simulink model "QBot2e_Path_Planning_Motion_Control"  (Simulink 10.1)
settings: Solver=ode1  StartTime=0.0  StopTime=inf  FixedStep=0.01  RelTol=1e-3  EnableMultiTasking=on
undefined symbols (not defined in the file or in its folder): HIL
libraries: quarc_library x8
settings Model: Creator=drmadill  LastModifiedBy=78253  SimulationMode=external  ExtModeTrigDuration=10000
settings SolverCC: PositivePriorityOrder=on
settings DataIOCC: LimitDataPoints=on  SignalLoggingSaveFormat=ModelDataLogs
settings OptimizationCC: ExpressionDepthLimit=2147483647  LifeSpan=auto
settings DebuggingCC: SolverPrmCheckMsg=warning  FcnCallInpInsideContextMsg=warning  StateNameClashWarn=warning
settings RTWCC: Description=QUARC Linux Raspberry Pi 3 Target  SystemTargetFile=quarc_linux_pi_3.tlc  TemplateMakefile=quarc_default_tmf
settings STFCustomTargetCC: TargetLibSuffix=.a  TargetPreCompLibLocation=C:\PROGRA~3\QUARC\lib\2018a\LINUX_~1\release  ConcurrentExecutionCompliant=on  SystemTargetFile=quarc_linux_pi_3.tlc
settings GRTTargetCC: TargetLibSuffix=.a  TargetPreCompLibLocation=C:\PROGRA~3\QUARC\lib\2018a\LINUX_~1\release  ParMdlRefBuildCompliant=off  CompOptLevelCompliant=off  MatFileLogging=off  CPPClassGenCompliant=off  UseToolchainInfoCompliant=off  ExtMode=on  ExtModeMexFile=quarc_comm  ExtModeMexArgs='-w -d /tmp -uri %u','tcpip://192.168.2.227:17001'
settings ConfigComp: CovSFcnEnable=off

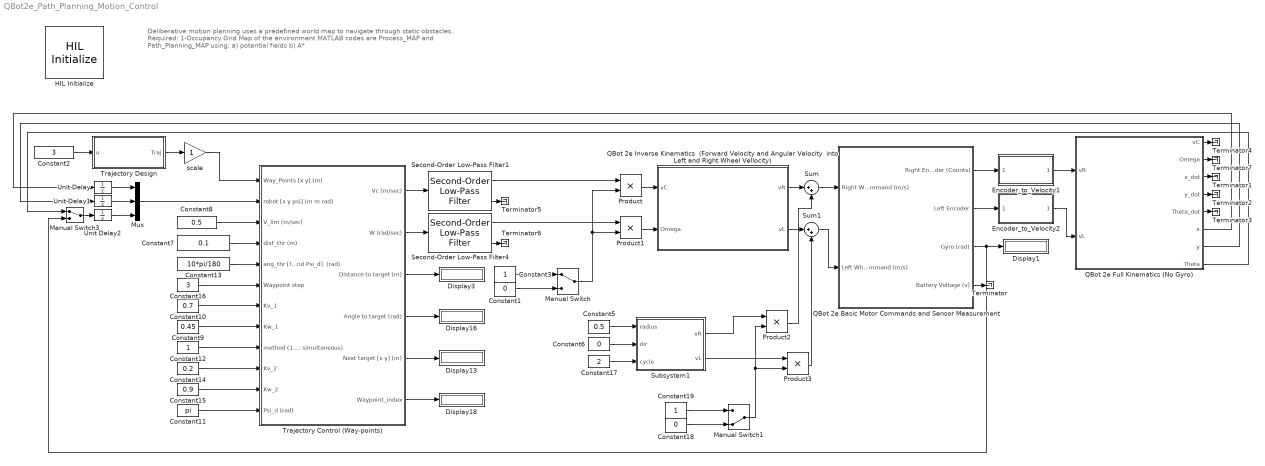
== system QBot2e_Path_Planning_Motion_Control ==
  note: Deliberative motion planning uses a predefined world map to navigate through static obstacles.
      |
      | Required:
      | 1-Occupancy Grid Map of the environment
      | MATLAB codes are Process_MAP and Path_Planning_MAP using:
      | a) potential fields
      | b) A*
  Constant1 : Constant  Value=0
  Constant10 : Constant  Value=0.7
  Constant11 : Constant  Value=pi
  Constant12 : Constant
  Constant13 : Constant  Value=10*pi/180
  Constant14 : Constant  Value=0.2
  Constant15 : Constant  Value=0.9
  Constant16 : Constant  Value=3
  Constant17 : Constant  Value=2
  Constant18 : Constant  Value=0
  Constant19 : Constant
  Constant2 : Constant  Value=3
  Constant3 : Constant
  Constant5 : Constant  Value=0.5
  Constant6 : Constant  Value=0
  Constant7 : Constant  Value=0.1
  Constant8 : Constant  Value=0.5
  Constant9 : Constant  Value=0.45
  Display{1,3,13,16,18} (5 alike) : Display
  Encoder_to_Velocity1 : Subsystem
  Encoder_to_Velocity2 : Subsystem
  HIL Initialize : quarc_library/Data Acquisition/Generic/Configuration/HIL Initialize  Priority=-99  object_name=HIL-1  board_type=qbot2e  board_number=0  board_options=pwm0_en=1;pwm0_pin=12;pwm1_en=1;pwm1_pin=13;  exclusive=off  active=off  hardware_clocks=[]  clock_modes=[]  initial_clock_frequencies=[]  set_clock_params_at_start=off  set_clock_params_at_switch_in=off  set_clock_frequencies_at_start=off  set_clock_frequencies_at_switch_in=off  analog_input_channels=[0:5]  analog_input_configurations=[]  analog_input_maximums=[16.5 3.3 3.3 3.3 3.3 3.3]  analog_input_minimums=[0 0 0 0 0 0]  set_analog_input_params_at_start=off  set_analog_input_params_at_switch_in=off  analog_output_channels=[]  analog_output_maximums=[]  analog_output_minimums=[]  initial_analog_outputs=[]  final_analog_outputs=[]  watchdog_analog_outputs=[]  set_analog_output_params_at_start=off  set_analog_output_params_at_switch_in=off  set_analog_outputs_at_start=off  set_analog_outputs_at_switch_in=off  set_analog_outputs_at_terminate=off  set_analog_outputs_at_switch_out=off  set_analog_outputs_on_watchdog=off  digital_input_channels=[28:58]  digital_output_channels=[28:31]  digital_output_configuration=[]  initial_digital_outputs=[0]  final_digital_outputs=[0]  watchdog_digital_outputs=[]  set_digital_output_params_at_start=off  set_digital_output_params_at_switch_in=off  set_digital_outputs_at_start=on  set_digital_outputs_at_switch_in=off  set_digital_outputs_at_terminate=on  set_digital_outputs_at_switch_out=off  set_digital_outputs_on_watchdog=off  encoder_channels=[0:1]  quadrature=[4]  encoder_filter_frequency=[]  initial_encoder_counts=[0]  set_encoder_params_at_start=on  set_encoder_params_at_switch_in=off  set_encoder_counts_at_start=on  set_encoder_counts_at_switch_in=off  pwm_channels=[0:1]  pwm_modes=0  pwm_frequency=100e6 / 4095  pwm_configuration=[0]  pwm_alignment=[0]  pwm_polarity=[1]  pwm_leading_deadband=[]  pwm_trailing_deadband=[]  initial_pwm_outputs=[0]  final_pwm_outputs=[0]  watchdog_pwm_outputs=[]  set_pwm_params_at_start=on  set_pwm_params_at_switch_in=off  set_pwm_outputs_at_start=on  set_pwm_outputs_at_switch_in=off  set_pwm_outputs_at_terminate=on  set_pwm_outputs_at_switch_out=off  set_pwm_outputs_on_watchdog=off  other_output_channels=[2000:2001 14000 16000]  initial_other_outputs=[0 0 0 7]  final_other_outputs=[0 0 0 7]  watchdog_other_outputs=[]  set_other_outputs_at_start=on  set_other_outputs_at_switch_in=off  set_other_outputs_at_terminate=on  set_other_outputs_at_switch_out=off  set_other_outputs_on_watchdog=off
  Manual Switch : ManualSwitch
  Manual Switch1 : ManualSwitch  CurrentSetting=0
  Manual Switch3 : ManualSwitch
  Mux : Mux  Inputs=[1 1 1]
  Product{,1..3} (4 alike) : Product  RndMeth=Zero
  QBot 2e Basic Motor Commands and Sensor Measurement : Subsystem
  QBot 2e Full Kinematics (No Gyro) : Subsystem
  QBot 2e Inverse Kinematics  (Forward Velocity and Angular Velocity  into Left and Right Wheel Vellocity) : Subsystem
  Second-Order Low-Pass Filter1 : quarc_library/Continuous/Second-Order Low-Pass Filter  params_source=Internal (dialog parameters)  input_width=30  input_zeta=1  input_init=0
  Second-Order Low-Pass Filter4 : quarc_library/Continuous/Second-Order Low-Pass Filter  params_source=Internal (dialog parameters)  input_width=60  input_zeta=1  input_init=0
  Subsystem1 : Subsystem
  Sum : Sum  Inputs=|++
  Sum1 : Sum  Inputs=|++
  Terminator{,1..7} (8 alike) : Terminator
  Trajectory Control (Way-points) : Subsystem
  Trajectory Design : Subsystem
  Unit Delay : UnitDelay  SampleTime=-1  HasFrameUpgradeWarning=on
  Unit Delay1 : UnitDelay  SampleTime=-1  HasFrameUpgradeWarning=on
  Unit Delay2 : UnitDelay  SampleTime=-1  HasFrameUpgradeWarning=on
  scale : Gain
  wires:
  Constant3/1 -> Manual Switch/1
  Constant1/1 -> Manual Switch/2
  QBot 2e Basic Motor Commands and Sensor Measurement/1(Right Encoder (Counts)) -> Encoder_to_Velocity1/1(Encoder)
  QBot 2e Basic Motor Commands and Sensor Measurement/2(Left Encoder) -> Encoder_to_Velocity2/1(Encoder)
  QBot 2e Basic Motor Commands and Sensor Measurement/3(Gyro (rad)) -> Display1/1, Manual Switch3/2
  QBot 2e Full Kinematics (No Gyro)/8(Theta) -> Manual Switch3/1
  Encoder_to_Velocity1/1(Velocity) -> QBot 2e Full Kinematics (No Gyro)/1(vR)
  Encoder_to_Velocity2/1(Velocity) -> QBot 2e Full Kinematics (No Gyro)/2(vL)
  Second-Order Low-Pass Filter1/1 -> Product/1
  Second-Order Low-Pass Filter4/1 -> Product1/1
  Product/1 -> QBot 2e Inverse Kinematics  (Forward Velocity and Angular Velocity  into Left and Right Wheel Vellocity)/1(vC)
  Product1/1 -> QBot 2e Inverse Kinematics  (Forward Velocity and Angular Velocity  into Left and Right Wheel Vellocity)/2(Omega)
  Manual Switch/1 -> Product/2, Product1/2
  QBot 2e Full Kinematics (No Gyro)/3(x_dot) -> Terminator1/1
  QBot 2e Full Kinematics (No Gyro)/4(y_dot) -> Terminator2/1
  QBot 2e Full Kinematics (No Gyro)/5(Theta_dot) -> Terminator3/1
  Constant8/1 -> Trajectory Control (Way-points)/3(V_lim (m/sec))
  Constant7/1 -> Trajectory Control (Way-points)/4(dist_thr (m))
  Constant13/1 -> Trajectory Control (Way-points)/5(ang_thr [for method 1 and Psi_d]  (rad))
  Constant16/1 -> Trajectory Control (Way-points)/6(Waypoint step)
  Trajectory Control (Way-points)/3(Distance to target (m)) -> Display3/1
  Mux/1 -> Trajectory Control (Way-points)/2(robot [x y psi] (m m rad))
  Unit Delay/1 -> Mux/1
  Unit Delay1/1 -> Mux/2
  Unit Delay2/1 -> Mux/3
  Constant10/1 -> Trajectory Control (Way-points)/7(Kv_1)
  Constant9/1 -> Trajectory Control (Way-points)/8(Kw_1)
  Trajectory Control (Way-points)/4(Angle to target (rad)) -> Display16/1
  scale/1 -> Trajectory Control (Way-points)/1(Way_Points [x y] (m))
  Trajectory Control (Way-points)/1(Vc (m/sec)) -> Second-Order Low-Pass Filter1/1
  Trajectory Control (Way-points)/2(W (rad/sec)) -> Second-Order Low-Pass Filter4/1
  Manual Switch3/1 -> Unit Delay2/1
  Trajectory Control (Way-points)/5(Next target [x y] (m)) -> Display13/1
  Constant14/1 -> Trajectory Control (Way-points)/10(Kv_2)
  Constant15/1 -> Trajectory Control (Way-points)/11(Kw_2)
  Constant12/1 -> Trajectory Control (Way-points)/9("method (1: sequential, 2: simultaneous)")
  Constant11/1 -> Trajectory Control (Way-points)/12(Psi_d (rad))
  Trajectory Control (Way-points)/6(Waypoint_index) -> Display18/1
  QBot 2e Full Kinematics (No Gyro)/6(x) -> Unit Delay/1
  QBot 2e Full Kinematics (No Gyro)/7(y) -> Unit Delay1/1
  Second-Order Low-Pass Filter1/2 -> Terminator5/1
  Second-Order Low-Pass Filter4/2 -> Terminator6/1
  QBot 2e Full Kinematics (No Gyro)/1(vC) -> Terminator4/1
  QBot 2e Full Kinematics (No Gyro)/2(Omega) -> Terminator7/1
  QBot 2e Basic Motor Commands and Sensor Measurement/4(Battery Voltage (v)) -> Terminator/1
  QBot 2e Inverse Kinematics  (Forward Velocity and Angular Velocity  into Left and Right Wheel Vellocity)/2(vL) -> Sum1/1
  QBot 2e Inverse Kinematics  (Forward Velocity and Angular Velocity  into Left and Right Wheel Vellocity)/1(vR) -> Sum/1
  Sum/1 -> QBot 2e Basic Motor Commands and Sensor Measurement/1(Right Wheel Command (m/s))
  Sum1/1 -> QBot 2e Basic Motor Commands and Sensor Measurement/2(Left Wheel Command (m/s))
  Constant5/1 -> Subsystem1/1(radius)
  Constant6/1 -> Subsystem1/2(dir)
  Constant17/1 -> Subsystem1/3(cycle)
  Constant18/1 -> Manual Switch1/2
  Constant19/1 -> Manual Switch1/1
  Manual Switch1/1 -> Product3/2, Product2/2
  Subsystem1/1(vR) -> Product2/1
  Subsystem1/2(vL) -> Product3/1
  Product2/1 -> Sum/2
  Product3/1 -> Sum1/2
  Constant2/1 -> Trajectory Design/1(u)
  Trajectory Design/1(Traj) -> scale/1

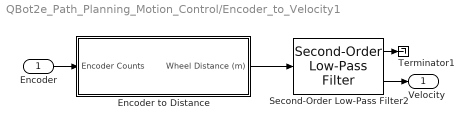
== system QBot2e_Path_Planning_Motion_Control/Encoder_to_Velocity1 ==
  Encoder : Inport
  Encoder to Distance : Subsystem
  Second-Order Low-Pass Filter2 : quarc_library/Continuous/Second-Order Low-Pass Filter  params_source=Internal (dialog parameters)  input_width=10  input_zeta=1  input_init=0
  Terminator1 : Terminator
  Velocity : Outport  VectorParamsAs1DForOutWhenUnconnected=off
  wires:
  Second-Order Low-Pass Filter2/1 -> Terminator1/1
  Encoder to Distance/1(Wheel Distance (m)) -> Second-Order Low-Pass Filter2/1
  Encoder/1 -> Encoder to Distance/1(Encoder Counts)
  Second-Order Low-Pass Filter2/2 -> Velocity/1

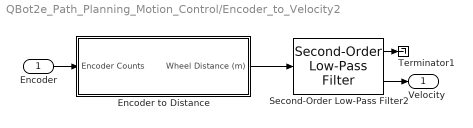
== system QBot2e_Path_Planning_Motion_Control/Encoder_to_Velocity2 ==
  Encoder : Inport
  Encoder to Distance : Subsystem
  Second-Order Low-Pass Filter2 : quarc_library/Continuous/Second-Order Low-Pass Filter  params_source=Internal (dialog parameters)  input_width=10  input_zeta=1  input_init=0
  Terminator1 : Terminator
  Velocity : Outport  VectorParamsAs1DForOutWhenUnconnected=off
  wires:
  Second-Order Low-Pass Filter2/2 -> Velocity/1
  Encoder/1 -> Encoder to Distance/1(Encoder Counts)
  Encoder to Distance/1(Wheel Distance (m)) -> Second-Order Low-Pass Filter2/1
  Second-Order Low-Pass Filter2/1 -> Terminator1/1

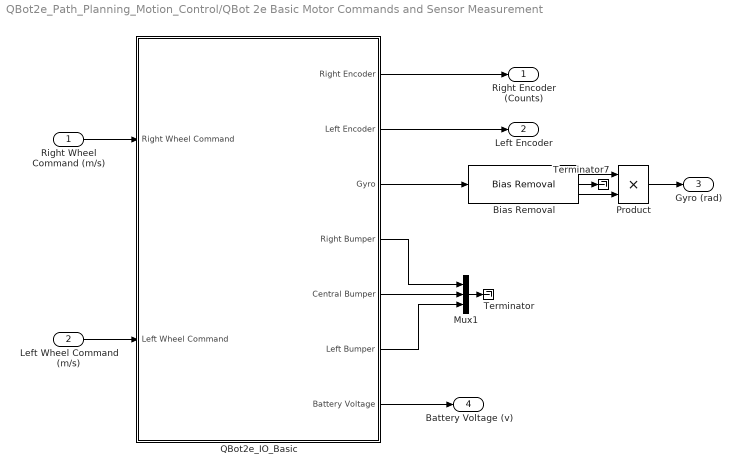
== system QBot2e_Path_Planning_Motion_Control/QBot 2e Basic Motor Commands and Sensor Measurement ==
  Right Wheel Command (m/s) : Inport
  Left Wheel Command (m/s) : Inport  Port=2
  Bias Removal : quarc_library/Discrete/Bias Removal  start_time=3  end_time=4  switch_id=0  sample_time=qc_get_step_size
      settings: SourceProductName=QUARC Targets
  Mux1 : Mux  Inputs=3
  Product : Product  RndMeth=Zero
  QBot2e_IO_Basic : Subsystem
  Terminator : Terminator
  Terminator7 : Terminator
  Right Encoder (Counts) : Outport  VectorParamsAs1DForOutWhenUnconnected=off
  Left Encoder : Outport  Port=2  VectorParamsAs1DForOutWhenUnconnected=off
  Gyro (rad) : Outport  Port=3  VectorParamsAs1DForOutWhenUnconnected=off
  Battery Voltage (v) : Outport  Port=4  VectorParamsAs1DForOutWhenUnconnected=off
  wires:
  QBot2e_IO_Basic/4(Right Bumper) -> Mux1/1
  QBot2e_IO_Basic/5(Central Bumper) -> Mux1/2
  QBot2e_IO_Basic/6(Left Bumper) -> Mux1/3
  Right Wheel Command (m/s)/1 -> QBot2e_IO_Basic/1(Right Wheel Command)
  Left Wheel Command (m/s)/1 -> QBot2e_IO_Basic/2(Left Wheel Command)
  QBot2e_IO_Basic/1(Right Encoder) -> Right Encoder (Counts)/1
  QBot2e_IO_Basic/2(Left Encoder) -> Left Encoder/1
  QBot2e_IO_Basic/7(Battery Voltage) -> Battery Voltage (v)/1
  Bias Removal/2 -> Terminator7/1
  Bias Removal/1 -> Product/1
  Bias Removal/3 -> Product/2
  Product/1 -> Gyro (rad)/1
  QBot2e_IO_Basic/3(Gyro) -> Bias Removal/1
  Mux1/1 -> Terminator/1

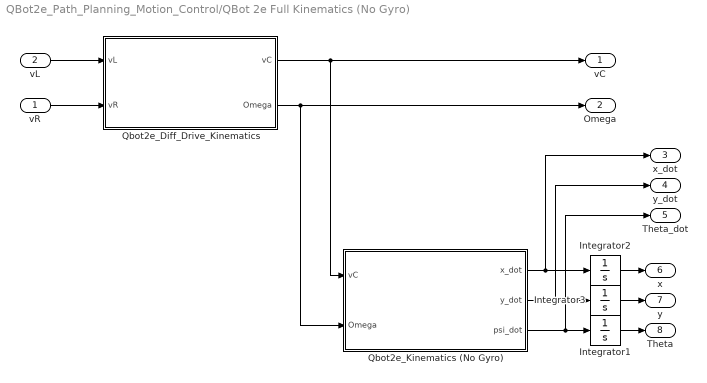
== system QBot2e_Path_Planning_Motion_Control/QBot 2e Full Kinematics (No Gyro) ==
  vR : Inport
  vL : Inport  Port=2
  Integrator1 : Integrator
  Integrator2 : Integrator
  Integrator3 : Integrator
  Qbot2e_Diff_Drive_Kinematics : Subsystem
  Qbot2e_Kinematics (No Gyro) : Subsystem
  vC : Outport  VectorParamsAs1DForOutWhenUnconnected=off
  Omega : Outport  Port=2  VectorParamsAs1DForOutWhenUnconnected=off
  x_dot : Outport  Port=3  VectorParamsAs1DForOutWhenUnconnected=off
  y_dot : Outport  Port=4  VectorParamsAs1DForOutWhenUnconnected=off
  Theta_dot : Outport  Port=5  VectorParamsAs1DForOutWhenUnconnected=off
  x : Outport  Port=6  VectorParamsAs1DForOutWhenUnconnected=off
  y : Outport  Port=7  VectorParamsAs1DForOutWhenUnconnected=off
  Theta : Outport  Port=8  VectorParamsAs1DForOutWhenUnconnected=off
  wires:
  Integrator1/1 -> Theta/1
  Qbot2e_Kinematics (No Gyro)/3(psi_dot) -> Theta_dot/1, Integrator1/1
  Qbot2e_Kinematics (No Gyro)/1(x_dot) -> x_dot/1, Integrator2/1
  Qbot2e_Kinematics (No Gyro)/2(y_dot) -> y_dot/1, Integrator3/1
  Qbot2e_Diff_Drive_Kinematics/1(vC) -> Qbot2e_Kinematics (No Gyro)/1(vC), vC/1
  vL/1 -> Qbot2e_Diff_Drive_Kinematics/1(vL)
  vR/1 -> Qbot2e_Diff_Drive_Kinematics/2(vR)
  Integrator2/1 -> x/1
  Integrator3/1 -> y/1
  Qbot2e_Diff_Drive_Kinematics/2(Omega) -> Qbot2e_Kinematics (No Gyro)/2(Omega), Omega/1

== system QBot2e_Path_Planning_Motion_Control/QBot 2e Inverse Kinematics  (Forward Velocity and Angular Velocity  into Left and Right Wheel Vellocity) ==
  vC : Inport
  Omega : Inport  Port=2
  Qbot2e_Inverse_Kinematics  (Forward Velocity and Angular Velocity into Left and Right Wheel Vellocity) : MATLAB Function  TreatAsAtomicUnit=on
  vR : Outport  VectorParamsAs1DForOutWhenUnconnected=off
  vL : Outport  Port=2  VectorParamsAs1DForOutWhenUnconnected=off
  wires:
  Qbot2e_Inverse_Kinematics  (Forward Velocity and Angular Velocity into Left and Right Wheel Vellocity)/2(vL) -> vL/1
  Omega/1 -> Qbot2e_Inverse_Kinematics  (Forward Velocity and Angular Velocity into Left and Right Wheel Vellocity)/2(Omega)
  Qbot2e_Inverse_Kinematics  (Forward Velocity and Angular Velocity into Left and Right Wheel Vellocity)/1(vR) -> vR/1
  vC/1 -> Qbot2e_Inverse_Kinematics  (Forward Velocity and Angular Velocity into Left and Right Wheel Vellocity)/1(vC)

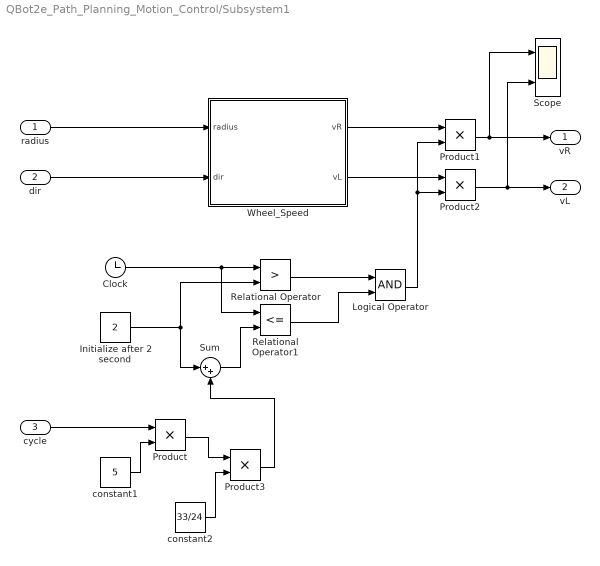
== system QBot2e_Path_Planning_Motion_Control/Subsystem1 ==
  radius : Inport
  dir : Inport  Port=2
  cycle : Inport  Port=3
  Clock : Clock
  Initialize after 2 second : Constant  Value=2
  Logical Operator : Logic  AllPortsSameDT=off  OutDataTypeStr=boolean
  Product{,1..3} (4 alike) : Product
  Relational Operator : RelationalOperator  Operator=>  OutDataTypeStr=boolean  RndMeth=Simplest
  Relational Operator1 : RelationalOperator  Operator=<=  OutDataTypeStr=boolean  RndMeth=Simplest
  Scope : Scope  NumInputPorts=2
  Sum : Sum  Inputs=|++
  Wheel_Speed : MATLAB Function  TreatAsAtomicUnit=on
  constant1 : Constant  Value=5
  constant2 : Constant  Value=33/24
  vR : Outport
  vL : Outport  Port=2
  wires:
  Sum/1 -> Relational Operator1/2
  Clock/1 -> Relational Operator1/1, Relational Operator/1
  Product2/1 -> Scope/2, vL/1
  Product1/1 -> Scope/1, vR/1
  Wheel_Speed/2(vL) -> Product2/1
  Relational Operator1/1 -> Logical Operator/2
  dir/1 -> Wheel_Speed/2(dir)
  cycle/1 -> Product/1
  Relational Operator/1 -> Logical Operator/1
  constant1/1 -> Product/2
  radius/1 -> Wheel_Speed/1(radius)
  Logical Operator/1 -> Product2/2, Product1/2
  Initialize after 2 second/1 -> Sum/1, Relational Operator/2
  Wheel_Speed/1(vR) -> Product1/1
  Product/1 -> Product3/1
  constant2/1 -> Product3/2
  Product3/1 -> Sum/2

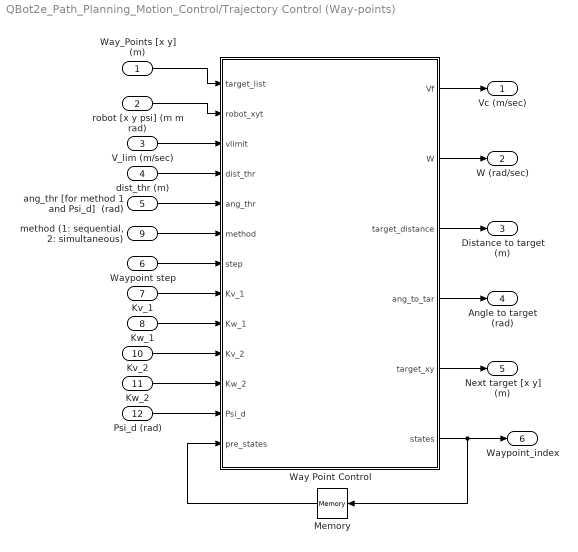
== system QBot2e_Path_Planning_Motion_Control/Trajectory Control (Way-points) ==
  Way_Points [x y] (m) : Inport
  robot [x y psi] (m m rad) : Inport  Port=2
  V_lim (m/sec) : Inport  Port=3
  dist_thr (m) : Inport  Port=4
  ang_thr [for method 1 and Psi_d]  (rad) : Inport  Port=5
  Waypoint step : Inport  Port=6
  Kv_1 : Inport  Port=7
  Kw_1 : Inport  Port=8
  "method (1: sequential, 2: simultaneous)" : Inport  Port=9
  Kv_2 : Inport  Port=10
  Kw_2 : Inport  Port=11
  Psi_d (rad) : Inport  Port=12
  Memory : Memory  InitialCondition=[0]
  Way Point Control : MATLAB Function  TreatAsAtomicUnit=on
  Vc (m/sec) : Outport  VectorParamsAs1DForOutWhenUnconnected=off
  W (rad/sec) : Outport  Port=2  VectorParamsAs1DForOutWhenUnconnected=off
  Distance to target (m) : Outport  Port=3  VectorParamsAs1DForOutWhenUnconnected=off
  Angle to target (rad) : Outport  Port=4  VectorParamsAs1DForOutWhenUnconnected=off
  Next target [x y] (m) : Outport  Port=5  VectorParamsAs1DForOutWhenUnconnected=off
  Waypoint_index : Outport  Port=6  VectorParamsAs1DForOutWhenUnconnected=off
  wires:
  Memory/1 -> Way Point Control/13(pre_states)
  Way Point Control/6(states) -> Memory/1, Waypoint_index/1
  Way_Points [x y] (m)/1 -> Way Point Control/1(target_list)
  Way Point Control/1(Vf) -> Vc (m/sec)/1
  robot [x y psi] (m m rad)/1 -> Way Point Control/2(robot_xyt)
  V_lim (m/sec)/1 -> Way Point Control/3(vlimit)
  Way Point Control/2(W) -> W (rad/sec)/1
  dist_thr (m)/1 -> Way Point Control/4(dist_thr)
  Way Point Control/3(target_distance) -> Distance to target (m)/1
  ang_thr [for method 1 and Psi_d]  (rad)/1 -> Way Point Control/5(ang_thr)
  Way Point Control/4(ang_to_tar) -> Angle to target (rad)/1
  Waypoint step/1 -> Way Point Control/7(step)
  Kv_1/1 -> Way Point Control/8(Kv_1)
  Way Point Control/5(target_xy) -> Next target [x y] (m)/1
  Kw_1/1 -> Way Point Control/9(Kw_1)
  "method (1: sequential, 2: simultaneous)"/1 -> Way Point Control/6(method)
  Kv_2/1 -> Way Point Control/10(Kv_2)
  Kw_2/1 -> Way Point Control/11(Kw_2)
  Psi_d (rad)/1 -> Way Point Control/12(Psi_d)

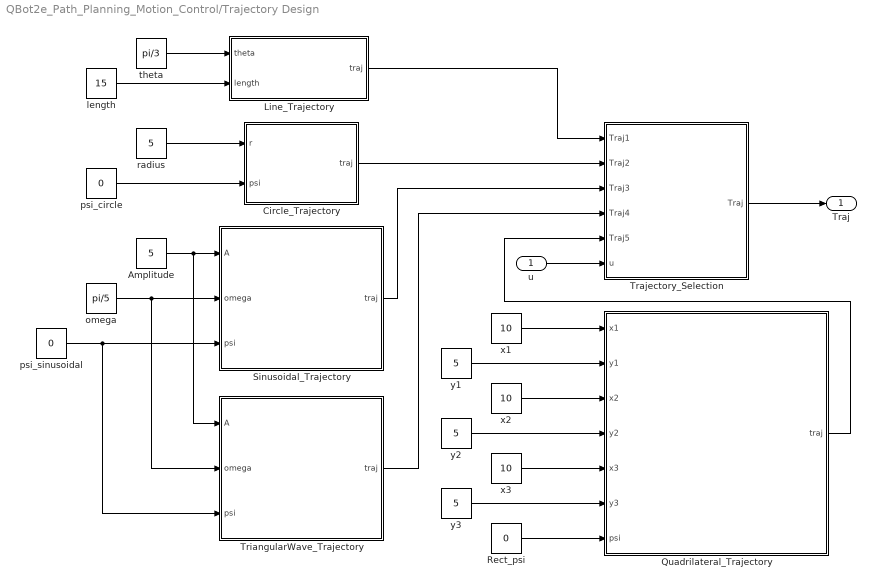
== system QBot2e_Path_Planning_Motion_Control/Trajectory Design ==
  u : Inport
  Amplitude : Constant  Value=5
  Circle_Trajectory : MATLAB Function  TreatAsAtomicUnit=on
  Line_Trajectory : MATLAB Function  TreatAsAtomicUnit=on
  "Quadrilateral_Trajectory " : MATLAB Function  TreatAsAtomicUnit=on
  Rect_psi : Constant  Value=0
  Sinusoidal_Trajectory : MATLAB Function  TreatAsAtomicUnit=on
  Trajectory_Selection : MATLAB Function  TreatAsAtomicUnit=on
  TriangularWave_Trajectory : MATLAB Function  TreatAsAtomicUnit=on
  length : Constant  Value=15
  omega : Constant  Value=pi/5
  psi_circle : Constant  Value=0
  psi_sinusoidal : Constant  Value=0
  radius : Constant  Value=5
  theta : Constant  Value=pi/3
  x1 : Constant  Value=10
  x2 : Constant  Value=10
  x3 : Constant  Value=10
  y1 : Constant  Value=5
  y2 : Constant  Value=5
  y3 : Constant  Value=5
  Traj : Outport
  wires:
  Trajectory_Selection/1(Traj) -> Traj/1
  Circle_Trajectory/1(traj) -> Trajectory_Selection/2(Traj2)
  psi_sinusoidal/1 -> TriangularWave_Trajectory/3(psi), Sinusoidal_Trajectory/3(psi)
  Amplitude/1 -> Sinusoidal_Trajectory/1(A), TriangularWave_Trajectory/1(A)
  omega/1 -> TriangularWave_Trajectory/2(omega), Sinusoidal_Trajectory/2(omega)
  Sinusoidal_Trajectory/1(traj) -> Trajectory_Selection/3(Traj3)
  theta/1 -> Line_Trajectory/1(theta)
  length/1 -> Line_Trajectory/2(length)
  psi_circle/1 -> Circle_Trajectory/2(psi)
  radius/1 -> Circle_Trajectory/1(r)
  Line_Trajectory/1(traj) -> Trajectory_Selection/1(Traj1)
  u/1 -> Trajectory_Selection/6(u)
  x1/1 -> "Quadrilateral_Trajectory "/1(x1)
  y1/1 -> "Quadrilateral_Trajectory "/2(y1)
  Rect_psi/1 -> "Quadrilateral_Trajectory "/7(psi)
  x2/1 -> "Quadrilateral_Trajectory "/3(x2)
  y2/1 -> "Quadrilateral_Trajectory "/4(y2)
  x3/1 -> "Quadrilateral_Trajectory "/5(x3)
  y3/1 -> "Quadrilateral_Trajectory "/6(y3)
  "Quadrilateral_Trajectory "/1(traj) -> Trajectory_Selection/5(Traj5)
  TriangularWave_Trajectory/1(traj) -> Trajectory_Selection/4(Traj4)

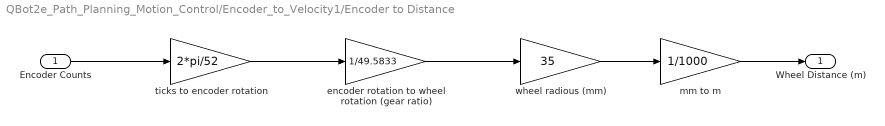
== system QBot2e_Path_Planning_Motion_Control/Encoder_to_Velocity1/Encoder to Distance ==
  Encoder Counts : Inport
  " encoder rotation to wheel rotation (gear ratio)" : Gain  Gain=1/49.5833
  mm to m : Gain  Gain=1/1000
  ticks to encoder rotation : Gain  Gain=2*pi/52
  wheel radious (mm) : Gain  Gain=35
  Wheel Distance (m) : Outport  VectorParamsAs1DForOutWhenUnconnected=off
  wires:
  Encoder Counts/1 -> ticks to encoder rotation/1
  ticks to encoder rotation/1 -> " encoder rotation to wheel rotation (gear ratio)"/1
  " encoder rotation to wheel rotation (gear ratio)"/1 -> wheel radious (mm)/1
  wheel radious (mm)/1 -> mm to m/1
  mm to m/1 -> Wheel Distance (m)/1

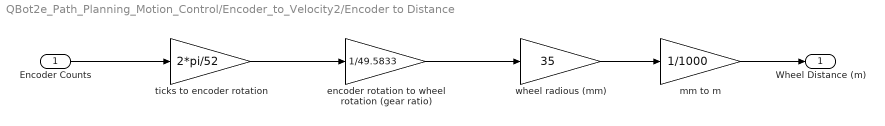
== system QBot2e_Path_Planning_Motion_Control/Encoder_to_Velocity2/Encoder to Distance ==
  Encoder Counts : Inport
  " encoder rotation to wheel rotation (gear ratio)" : Gain  Gain=1/49.5833
  mm to m : Gain  Gain=1/1000
  ticks to encoder rotation : Gain  Gain=2*pi/52
  wheel radious (mm) : Gain  Gain=35
  Wheel Distance (m) : Outport  VectorParamsAs1DForOutWhenUnconnected=off
  wires:
  mm to m/1 -> Wheel Distance (m)/1
  wheel radious (mm)/1 -> mm to m/1
  " encoder rotation to wheel rotation (gear ratio)"/1 -> wheel radious (mm)/1
  ticks to encoder rotation/1 -> " encoder rotation to wheel rotation (gear ratio)"/1
  Encoder Counts/1 -> ticks to encoder rotation/1

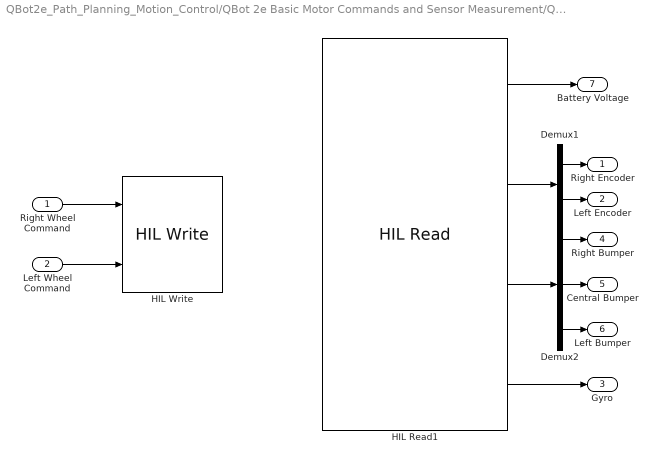
== system QBot2e_Path_Planning_Motion_Control/QBot 2e Basic Motor Commands and Sensor Measurement/QBot2e_IO_Basic ==
  Right Wheel Command : Inport
  Left Wheel Command : Inport  Port=2
  Demux1 : Demux  Outputs=2
  Demux2 : Demux  Outputs=3
  HIL Read1 : quarc_library/Data Acquisition/Generic/Immediate I//O/HIL Read  object_name=HIL-1  analog_channels=[0]  encoder_channels=[0:1]  digital_channels=[28:30]  other_channels=[1002]  sample_time=qc_get_step_size  active=on  vector_output=on  data_type_mode=Inherit via back propagation  encoder_data_type=double  digital_data_type=boolean
  HIL Write : quarc_library/Data Acquisition/Generic/Immediate I//O/HIL Write  object_name=HIL-1  analog_channels=[]  pwm_channels=[]  digital_channels=[]  other_channels=[2000:2001]  sample_time=-1  active=on  vector_input=off
  Right Encoder : Outport  VectorParamsAs1DForOutWhenUnconnected=off
  Left Encoder : Outport  Port=2  VectorParamsAs1DForOutWhenUnconnected=off
  Gyro : Outport  Port=3  VectorParamsAs1DForOutWhenUnconnected=off
  Right Bumper : Outport  Port=4  VectorParamsAs1DForOutWhenUnconnected=off
  Central Bumper : Outport  Port=5  VectorParamsAs1DForOutWhenUnconnected=off
  Left Bumper : Outport  Port=6  VectorParamsAs1DForOutWhenUnconnected=off
  Battery Voltage : Outport  Port=7  VectorParamsAs1DForOutWhenUnconnected=off
  wires:
  HIL Read1/1 -> Battery Voltage/1
  HIL Read1/3 -> Demux2/1
  HIL Read1/4 -> Gyro/1
  Demux1/1 -> Right Encoder/1
  Demux1/2 -> Left Encoder/1
  Right Wheel Command/1 -> HIL Write/1
  Left Wheel Command/1 -> HIL Write/2
  HIL Read1/2 -> Demux1/1
  Demux2/1 -> Right Bumper/1
  Demux2/2 -> Central Bumper/1
  Demux2/3 -> Left Bumper/1

== system QBot2e_Path_Planning_Motion_Control/QBot 2e Full Kinematics (No Gyro)/Qbot2e_Diff_Drive_Kinematics ==
  vL : Inport
  vR : Inport  Port=2
  Qbot2_Diff_Drive_Kinematics : MATLAB Function  TreatAsAtomicUnit=on
  vC : Outport  VectorParamsAs1DForOutWhenUnconnected=off
  Omega : Outport  Port=2  VectorParamsAs1DForOutWhenUnconnected=off
  wires:
  vL/1 -> Qbot2_Diff_Drive_Kinematics/1(vL)
  Qbot2_Diff_Drive_Kinematics/1(vC) -> vC/1
  vR/1 -> Qbot2_Diff_Drive_Kinematics/2(vR)
  Qbot2_Diff_Drive_Kinematics/2(Omega) -> Omega/1

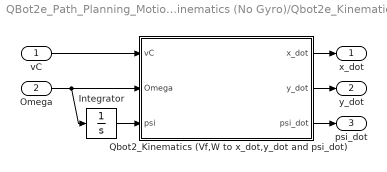
== system QBot2e_Path_Planning_Motion_Control/QBot 2e Full Kinematics (No Gyro)/Qbot2e_Kinematics (No Gyro) ==
  vC : Inport
  Omega : Inport  Port=2
  Integrator : Integrator
  Qbot2_Kinematics (Vf,W to x_dot,y_dot and psi_dot) : MATLAB Function  TreatAsAtomicUnit=on
  x_dot : Outport  VectorParamsAs1DForOutWhenUnconnected=off
  y_dot : Outport  Port=2  VectorParamsAs1DForOutWhenUnconnected=off
  psi_dot : Outport  Port=3  VectorParamsAs1DForOutWhenUnconnected=off
  wires:
  Qbot2_Kinematics (Vf,W to x_dot,y_dot and psi_dot)/3(psi_dot) -> psi_dot/1
  Integrator/1 -> Qbot2_Kinematics (Vf,W to x_dot,y_dot and psi_dot)/3(psi)
  vC/1 -> Qbot2_Kinematics (Vf,W to x_dot,y_dot and psi_dot)/1(vC)
  Qbot2_Kinematics (Vf,W to x_dot,y_dot and psi_dot)/1(x_dot) -> x_dot/1
  Omega/1 -> Integrator/1, Qbot2_Kinematics (Vf,W to x_dot,y_dot and psi_dot)/2(Omega)
  Qbot2_Kinematics (Vf,W to x_dot,y_dot and psi_dot)/2(y_dot) -> y_dot/1

== matlab function Trajectory Design/Circle_Trajectory ==
  data: traj output double; r input double; psi input double
function traj = Cir_Traj(r, psi)
% First we only care about the specific circle that satisfies
% x^2 + (y-r)^2 = r^2, where r is the radius of the circle.
% And in the polar coordinate system, it is:
% ρ = 2*r*sin(θ), where θ is between 0 and π.

% From the start point to the end point, there are N steps.
% Thus we divide π into N segments, that is, for the i th point sampled in
% the trajectory, its polar coordinate (ρi,θi) = (2*r*sin(θi), θi),
% where θi = (π/N)*(i-1).
% Finally, change the polar coordinate back to the Cartesian (xi, yi).

% Then, if the circle is rotated around the origin by ψ counterclockwise,
% we just do a coordinate transformation.

traj = zeros(20, 2);   % initialize

for i = 1 : 20
    theta_i = (pi/19) * (i-1);
    rou_i = 2 * r * sin(theta_i);
    px_t = rou_i * cos(theta_i);
    py_t = rou_i * sin(theta_i);
    % coordinate transformation when the circle is rotated by psi
    traj(i,1) = px_t * cos(psi) - py_t * sin(psi);
    traj(i,2) = px_t * sin(psi) + py_t * cos(psi);
end

== matlab function QBot 2e Full Kinematics (No Gyro)/Qbot2e_Diff_Drive_Kinematics/Qbot2_Diff_Drive_Kinematics ==
  data: vL input double; vC output double; vR input double; Omega output double
function [vC,Omega] = fcn(vL,vR)
%#codegen

d= 0.235;

vC=0.5*(vL+vR);
Omega=(1/d)*(vR-vL);

== matlab function QBot 2e Full Kinematics (No Gyro)/Qbot2e_Kinematics (No Gyro)/Qbot2_Kinematics (Vf,W to x_dot,y_dot and psi_dot) ==
  data: vC input double; x_dot output double; Omega input double; y_dot output double; psi input double; psi_dot output double
function [x_dot,y_dot,psi_dot] = fcn(vC,Omega,psi)
%#codegen


x_dot=cos(psi)*vC;
y_dot=sin(psi)*vC;
psi_dot= Omega;

== matlab function Trajectory Control (Way-points)/Way Point Control ==
  data: target_list input double; robot_xyt input double; vlimit input double; dist_thr input double; ang_thr input double; method input double; step input double; Kv_1 input double; Kw_1 input double; Kv_2 input double; Kw_2 input double; Psi_d input double; Vf output double; W output double; target_distance output double; ang_to_tar output double; target_xy output double; states output double; pre_states input double
function [Vf, W, target_distance, ang_to_tar, target_xy, states] = ...
    WaypointControl(target_list, robot_xyt, vlimit, ...
    dist_thr, ang_thr, method, step, Kv_1, Kw_1, Kv_2, Kw_2, Psi_d, pre_states)

% Initialize output variables

 Vf=0;
 W=0;
 finished_path_flag=0; 
 
 persistent Vf_1 end_flag;
 
 if isempty(Vf_1)
     Vf_1=0;
 end
 if isempty(end_flag)
    end_flag = 0;
 end
states = pre_states;



rx = robot_xyt(1);
ry = robot_xyt(2);
rtheta = check_angle(robot_xyt(3));
target_xy = [rx ry];
[n xy] = size(target_list);
if n==2 && xy==1
    target_xy = [target_list(1,1) target_list(2,1)];
    n = 1;
else
    for i=1:n
        if states(1) == i
            for j=1:xy
                target_xy(j) = target_list(i, j);
            end
        end
    end
end

tx = target_xy(1);
ty = target_xy(2);
target_distance = find_dist(rx, ry, tx, ty);
ang_to_tar= find_theta(rx, ry, rtheta, tx, ty);

if ((states(1) == n) && (target_distance <= dist_thr))  %|| states(1) == -1
% %        states(1) = -1;
       % right_vel = int16(0);
       % left_vel = int16(0);
%  %       target_distance = 0;
        Vf=0;
        W=0;
        
       if (end_flag == 1) && (target_distance <= dist_thr) % after all waypoints, psi will be adjusted to psi_d 
            [Vf, W] = ClosedLoop_Sequential(0, check_angle(check_angle(Psi_d)-check_angle(rtheta)), vlimit, ang_thr, dist_thr, Kv_1, Kw_1, Vf_1); 
             Vf_1=Vf;
       end
        
   
else
    
    if (target_distance <= dist_thr) && (end_flag==0)
            states(1) = pre_states(1) + step;%1;
      if( pre_states(1)>0 )      
         while (abs((target_list(states(1),1))-(target_list(pre_states(1),1)))<2*dist_thr) && (abs((target_list(states(1),2))-(target_list(pre_states(1),2)))<2*dist_thr)
             if (states(1)<=(n-step))
                 states(1) = states(1) + step;%1;
             else
                 states(1)=n;
             end
         end
      else
          states(1)=states(1)+step;
      end
         if states(1) >= n 
            states(1) = n;
            end_flag=1;
         end
        
               
  %  elseif (end_flag == 1) && (target_distance <= dist_thr) % after all waypoints, psi will be adjusted to psi_d 
  %          [Vf, W] = ClosedLoop_Sequential(0, check_angle(check_angle(Psi_d)-check_angle(rtheta)), vlimit, ang_thr, dist_thr, Kv_1, Kw_1, Vf_1); 
  %           Vf_1=Vf;
    else
        
        
            if method == 2
                [Vf, W] = ClosedLoop_Both(target_distance,  ang_to_tar, vlimit, Kv_2, Kw_2);    
            else
    %            [right_vel, left_vel] = rotate_and_go(ang_to_tar, vlimit, ang_thr);
                [Vf, W] = ClosedLoop_Sequential(target_distance,  ang_to_tar, vlimit, ang_thr, dist_thr, Kv_1, Kw_1, Vf_1); 
                Vf_1=Vf;
            end
                 
    end
end


return;

%--------------------------------------------------------------------------
function [y] = check_angle(x)
y = x;
if x > pi
    y = x - 2*pi;
elseif x < -pi
    y = x + 2*pi;
end
return;
% -------------------------------------------------------------------------
function dist = find_dist(rx, ry, tx, ty)
dist = sqrt((rx-tx)^2 + (ry-ty)^2);
return;
% -------------------------------------------------------------------------
function [theta]= find_theta(rx, ry, rtheta, tx, ty)

X = tx - rx;
Y = ty - ry;
theta = atan2(Y, X);
theta = check_angle(check_angle(theta)-check_angle(rtheta));

return;
% -------------------------------------------------------------------------

function [Vf, W] = ClosedLoop_Both(dist, theta, vlimit, Kv,Kw)

d = 0.23;
vmax = vlimit;
wmax = (2*vmax);
W = Kw*theta;

%if abs(theta)<pi
Vf = Kv*dist;
%else
%    Vf=0;
%end

w_sign = sign(W);
if abs(W) > wmax
    W = w_sign*wmax;
end
if abs(Vf)> vlimit
    Vf = abs(Vf)*vlimit;
end

return;

function [Vf, W] = ClosedLoop_Sequential(dist, theta, vlimit, ang_thr, dist_thr, Kv, Kw, Vf_1)

d = 0.23;
vmax = vlimit;
wmax = (2*vmax);

if (((abs(theta) > ang_thr))  && (Vf_1<0.01)) || (abs(theta) > 5*ang_thr) % once rotated, then moves. once started moving, it won't turn unless the heading is too off target or have reached the previous target.
        W=Kw*theta;
        Vf=0;
        if abs(W)> wmax
            W=sign(theta)*wmax;
        end
else
        Vf=Kv*dist;
       
        if abs(Vf)>vlimit
            Vf=sign(Vf)*vlimit;
        end
       % if (abs(theta) > 2*ang_thr)
       %   W=Kw*theta;
       %   Vf=0.4*Vf;
       % else
       W=0;
       % end
       % if abs(W)> wmax
       %     W=sign(theta)*wmax;
       % end
        
end

return;

%{
function [vr, vl] = solve_inv_kin(dist, theta, vlimit, delta_t)

d = 0.23;
vmax = vlimit(2);
wmax = (2*vmax)/d;
w = theta/delta_t;
w_sign = sign(w);
if abs(w) > wmax
    w = w_sign*wmax;
    vr = int16(round((d*w)/2));
    vl = int16(-vr);
else
    v = dist/delta_t;
    vr_tmp = (2*v + d*w)/2;
    vl_tmp = 2*v - vr_tmp;
    
    max_of_vrvl = abs(max(vr_tmp, vl_tmp));
    if max_of_vrvl > vmax
        vr_tmp = (vr_tmp/max_of_vrvl)*vmax;
        vl_tmp = (vl_tmp/max_of_vrvl)*vmax;
    end
    vr = int16(vr_tmp);
    vl = int16(vl_tmp);

end


return;
%}

%{
% -------------------------------------------------------------------------
function [vr, vl] = rotate_and_go(theta, vlimit, ang_thr)

if abs(theta) > ang_thr
    if theta >= 0
        vr = int16(vlimit(1));
        vl = int16(-vlimit(1));
    else
        vr = int16(-vlimit(1));
        vl = int16(vlimit(1));
    end
else
        vr = int16(vlimit(2));
        vl = int16(vlimit(2));
end

return;
% -------------------------------------------------------------------------
%}

== matlab function Trajectory Design/Line_Trajectory ==
  data: traj output double; theta input double; length input double
function traj = Line_Traj(theta, length)
% theta is the dip angle by the x-axis, thus the slope k = tan(theta).
% theta is radian instead of degree.

% length is the length of the line trajectory.

traj = zeros(20, 2);   % initialize

length_x = length * cos(theta);
length_y = length * sin(theta);

for i = 1 : 20
    traj(i,1) = length_x/20 * (i-1);
    traj(i,2) = length_y/20 * (i-1);
end

== matlab function Trajectory Design/Sinusoidal_Trajectory ==
  data: traj output double; A input double; omega input double; psi input double
function traj = Sin_Traj(A, omega, psi)
% We always and only focus on the sinusoidal curve whose phase is 0.

% First we only care about the sinusoidal curve that expands along the
% x-axis, that is, y = A * sin(ω*t).
% cycle is how many cycles we're going along the sinusoidal trajectory.
% Thus, the distance we're going along on the component of the x-axis is:
% dis_on_x = (2π/ω) * cycle.

% From the start point to the end point, there are N steps.
% Thus we divide dis_on_x into N segments, that is, for the i th point
% sampled in the trajectory, (xi, yi) = (xi, A*sin(omega*xi)),
% where xi = (dis_on_x/N)*(i-1).

% Then, if the circle is rotated around the origin by ψ counterclockwise,
% we just do a coordinate transformation.

traj = zeros(20, 2);   % initialize

T = 2*pi/omega;

for i = 1 : 20
    px_t = T/20 * i;
    py_t = A * sin(omega * px_t);
    % coordinate transformation when the circle is rotated by psi
    traj(i,1) = px_t * cos(psi) - py_t * sin(psi);
    traj(i,2) = px_t * sin(psi) + py_t * cos(psi);
end

== matlab function Trajectory Design/Trajectory_Selection ==
  data: Traj1 input double; Traj2 input double; Traj3 input double; Traj4 input double; Traj5 input double; u input double; Traj output double
function Traj = Traj_Sel( Traj1, Traj2, Traj3, Traj4, Traj5, u)
% Trajectory Selection
% Traj divided by 10 is for scaling

if u == 1
    Traj = Traj1/10;
elseif u == 2
    Traj = Traj2/10;
elseif u == 3
    Traj = Traj3/10;
elseif u == 4
    Traj = Traj4/10;
else
    Traj = Traj5/10;
end

== matlab function Subsystem1/Wheel_Speed ==
  data: radius input double; vR output double; dir input double; vL output double
% 作者：Syy
% 编辑日期：2020/12/29  
function [vR, vL] = Wheel_Speed(radius, dir)
% 该模块直接控制quanser机器人进行圆轨迹的跟踪
% 输入radius为圆的半径，输入dir为圆的方向（0为逆时针，1位顺时针）
 omega = 1.2547;    % 角速度
 d = 0.235;         % 小车直径
 vR = 0; vL = 0;
 if dir == 0
     vR = omega*(radius + d/2);
     vL = omega*(radius - d/2);
 elseif dir == 1
     vR = omega*(radius - d/2);
     vL = omega*(radius + d/2);
 end

== matlab function Trajectory Design/Quadrilateral_Trajectory  ==
  data: x1 input double; traj output double; y1 input double; x2 input double; y2 input double; x3 input double; y3 input double; psi input double
function traj = Quad_Traj(x1, y1, x2, y2, x3, y3, psi)
% The trajectory can be the four sides of any quadrilateral we want.

% This time we do not use N to divide the whole process into several steps.
% The only process is to determine the Cartesian coordinates of the four
% vertices. And we always set one of them as the origin (0,0).That is, we
% set the four vertices as (0,0), (x1,y1), (x2,y2), (x3,y3).

% Then, if the rectangle rotats around the origin by ψ counterclockwise,
% we just do a coordinate transformation.

traj = zeros(20, 2);   % initialize the coordinates of the four vertices

traj(5,1) = x1; traj(5,2) = y1;
traj(10,1) = x2; traj(10,2) = y2;
traj(15,1) = x3; traj(15,2) = y3;
traj(20,1) = 0; traj(20,2) = 0;

for i = 1 : 4
    traj(i,1) = x1/5 * i;
    traj(i,2) = y1/5 * i;
end

for i = 6 : 9
    traj(i,1) = x1 + (x2-x1)/5 * (i-5);
    traj(i,2) = y1 + (y2-y1)/5 * (i-5);
end

for i = 11 : 14
    traj(i,1) = x2 + (x3-x2)/5 * (i-5);
    traj(i,2) = y2 + (y3-y2)/5 * (i-5);
end

for i = 16 : 19
    traj(i,1) = x3 + (0-x3)/5 * (i-5);
    traj(i,2) = y3 + (0-y3)/5 * (i-5);
end

for i = 1 : 20
    px_t = traj(i,1);
    py_t = traj(i,2);
    % coordinate transformation when the circle is rotated by psi
    traj(i,1) = px_t * cos(psi) - py_t * sin(psi);
    traj(i,2) = px_t * sin(psi) + py_t * cos(psi);
end

== matlab function QBot 2e Inverse Kinematics (Forward Velocity and Angular Velocity into Left and Right Wheel Vellocity)/Qbot2e_Inverse_Kinematics (Forward Velocity and Angular Velocity into Left and Right Wheel Vellocity) ==
  data: vR output double; vL output double; vC input double; Omega input double
function [vR,vL] = fcn(vC , Omega)
%#codegen

d=0.235; 
% Eqn Based on the eqn 4.52 (W is the angular velocity)

vR = vC + Omega*d/2;
vL= vC - Omega*d/2;

== matlab function Trajectory Design/TriangularWave_Trajectory ==
  data: traj output double; A input double; omega input double; psi input double
function traj = TriWave_Traj(A, omega, psi)
% We always and only focus on the sinusoidal curve whose phase is 0.

% From the start point to the end point, there are N steps.
% Thus we divide dis_on_x into N segments, that is, for the i th point
% sampled in the trajectory.

% Then, if the circle is rotated around the origin by ψ counterclockwise,
% we just do a coordinate transformation.

traj = zeros(20, 2);   % initialize

T = 2 * pi / omega;
for i = 1 : 20
    traj(i,1) = (T/20) * i;
end

for i = 1 : 5
    traj(i,2) = A/5 * i;
end
for i = 6 : 10
    traj(i,2) = A - A/5*i;
end
for i = 11 : 15
    traj(i,2) = -A/5 * i;
end
for i = 16 : 20
    traj(i,2) = -A + A/5*i;
end

for i = 1 : 20
    px_t = traj(i,1);
    py_t = traj(i,2);
    % coordinate transformation when the circle is rotated by psi
    traj(i,1) = px_t * cos(psi) - py_t * sin(psi);
    traj(i,2) = px_t * sin(psi) + py_t * cos(psi);
end
